simulink model "racing_car1"  (R2013a)
settings: Solver=ode3  StartTime=0.0  StopTime=100  FixedStep=1/60  MaxStep=0.01  MinStep=0.001  RelTol=1e-3
settings Model: Creator=Administrator  LastModifiedBy=CeHao

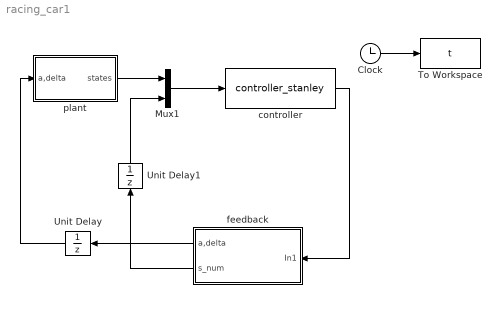
== system racing_car1 ==
  Clock : Clock
  Mux1 : Mux  Inputs=2
  To Workspace : ToWorkspace  VariableName=t  SampleTime=-1
  Unit Delay : UnitDelay  SampleTime=-1
  Unit Delay1 : UnitDelay  SampleTime=-1
  controller : S-Function  FunctionName=controller_stanley  Parameters=reference  EnableBusSupport=off
  feedback : Subsystem
  plant : Subsystem
  wires:
  Mux1/1 -> controller/1
  plant/1(states) -> Mux1/1
  Unit Delay/1 -> plant/1(a,delta)
  Unit Delay1/1 -> Mux1/2
  Clock/1 -> To Workspace/1
  controller/1 -> feedback/1(In1)
  feedback/1(a,delta) -> Unit Delay/1
  feedback/2(s_num) -> Unit Delay1/1

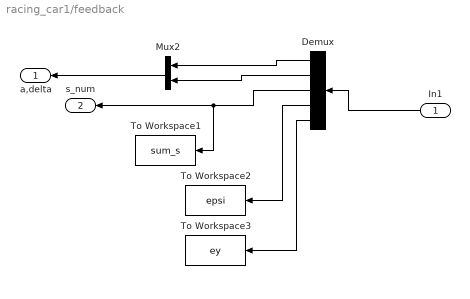
== system racing_car1/feedback ==
  In1 : Inport
  Demux : Demux  Outputs=5
  Mux2 : Mux  Inputs=2
  To Workspace1 : ToWorkspace  VariableName=sum_s  SampleTime=-1
  To Workspace2 : ToWorkspace  VariableName=epsi  SampleTime=-1
  To Workspace3 : ToWorkspace  VariableName=ey  SampleTime=-1
  a,delta : Outport
  s_num : Outport  Port=2
  wires:
  In1/1 -> Demux/1
  Demux/2 -> Mux2/2
  Demux/1 -> Mux2/1
  Mux2/1 -> a,delta/1
  Demux/3 -> To Workspace1/1, s_num/1
  Demux/4 -> To Workspace2/1
  Demux/5 -> To Workspace3/1

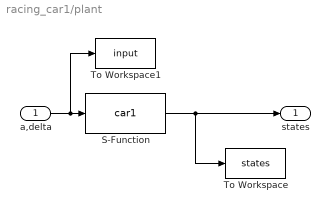
== system racing_car1/plant ==
  a,delta : Inport
  S-Function : S-Function  FunctionName=car1  Parameters=init  EnableBusSupport=off
  To Workspace : ToWorkspace  VariableName=states  SampleTime=-1
  To Workspace1 : ToWorkspace  VariableName=input  SampleTime=-1
  states : Outport
  wires:
  a,delta/1 -> To Workspace1/1, S-Function/1
  S-Function/1 -> states/1, To Workspace/1
